simulink model "cmvk"  (R2023b)
settings: Solver=VariableStepAuto  StartTime=0.0  StopTime=700  RelTol=1e-3
settings Model: Creator=Iustin  LastModifiedBy=Iustin

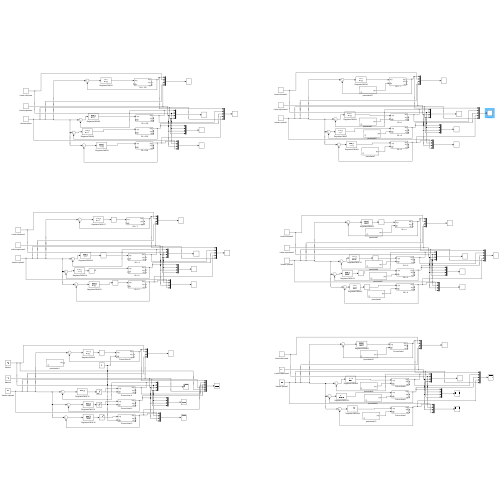
[thumbnail: Simulink's stored preview of the top-level diagram]
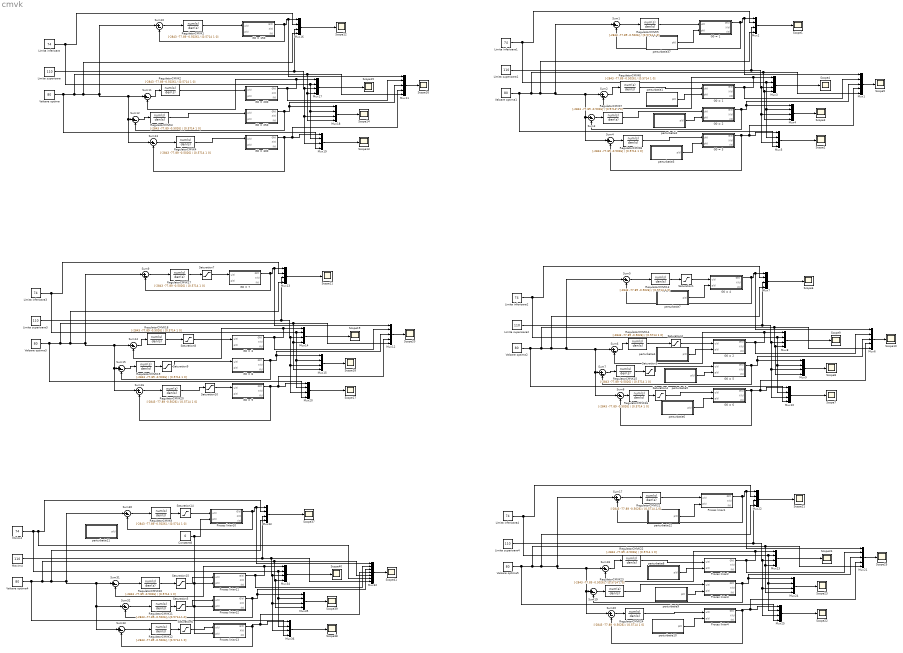
== system cmvk ==
  "  G0 = 1" : Subsystem  mask{p1=0.005, p2=0.017, p3=0.00000808, n=0.175, V=120, Gb=80, G0=100}
  "  G0 = 2" : Subsystem  mask{p1=0.005, p2=0.017, p3=0.00000808, n=0.175, V=120, Gb=80, G0=100}
  "  G0 = 200" : Subsystem  mask{p1=0.005, p2=0.017, p3=0.00000808, n=0.175, V=120, Gb=80, G0=200}
  "  G0 = 3" : Subsystem  mask{p1=0.005, p2=0.017, p3=0.00000808, n=0.175, V=120, Gb=80, G0=200}
  " G0 = 1" : Subsystem  mask{p1=0.005, p2=0.017, p3=0.00000808, n=0.175, V=120, Gb=80, G0=100}
  " G0 = 150" : Subsystem  mask{p1=0.005, p2=0.017, p3=0.00000808, n=0.175, V=120, Gb=80, G0=150}
  " G0 = 2" : Subsystem  mask{p1=0.005, p2=0.017, p3=0.00000808, n=0.175, V=120, Gb=80, G0=100}
  " G0 = 250" : Subsystem  mask{p1=0.005, p2=0.017, p3=0.00000808, n=0.175, V=120, Gb=80, G0=250}
  " G0 = 3" : Subsystem  mask{p1=0.005, p2=0.017, p3=0.00000808, n=0.175, V=120, Gb=80, G0=100}
  " G0 = 300" : Subsystem  mask{p1=0.005, p2=0.017, p3=0.00000808, n=0.175, V=120, Gb=80, G0=300}
  " G0 = 4" : Subsystem  mask{p1=0.005, p2=0.017, p3=0.00000808, n=0.175, V=120, Gb=80, G0=100}
  " G0 = 5" : Subsystem  mask{p1=0.005, p2=0.017, p3=0.00000808, n=0.175, V=120, Gb=80, G0=100}
  " G0 = 6" : Subsystem  mask{p1=0.005, p2=0.017, p3=0.00000808, n=0.175, V=120, Gb=80, G0=100}
  " G0 = 7" : Subsystem  mask{p1=0.005, p2=0.017, p3=0.00000808, n=0.175, V=120, Gb=80, G0=150}
  " G0 = 8" : Subsystem  mask{p1=0.005, p2=0.017, p3=0.00000808, n=0.175, V=120, Gb=80, G0=250}
  " G0 = 9" : Subsystem  mask{p1=0.005, p2=0.017, p3=0.00000808, n=0.175, V=120, Gb=80, G0=300}
  " Proces liniar1" : Subsystem  mask{p1=0.005, p2=0.017, p3=0.00000808, n=0.175, V=120, Gb=80, G0=150, Xb=0.0054}
  " Proces liniar10" : Subsystem  mask{p1=0.005, p2=0.017, p3=0.00000808, n=0.175, V=120, Gb=80, G0=150, Xb=0.0054}
  " Proces liniar11" : Subsystem  mask{p1=0.005, p2=0.017, p3=0.00000808, n=0.175, V=120, Gb=80, G0=200, Xb=0.0054}
  " Proces liniar12" : Subsystem  mask{p1=0.005, p2=0.017, p3=0.00000808, n=0.175, V=120, Gb=80, G0=250, Xb=0.0054}
  " Proces liniar13" : Subsystem  mask{p1=0.005, p2=0.017, p3=0.00000808, n=0.175, V=120, Gb=80, G0=300, Xb=0.0054}
  " Proces liniar2" : Subsystem  mask{p1=0.005, p2=0.017, p3=0.00000808, n=0.175, V=120, Gb=80, G0=150, Xb=0.0054}
  " Proces liniar3" : Subsystem  mask{p1=0.005, p2=0.017, p3=0.00000808, n=0.175, V=120, Gb=80, G0=150, Xb=0.0054}
  " Proces liniar4" : Subsystem  mask{p1=0.005, p2=0.017, p3=0.00000808, n=0.175, V=120, Gb=80, G0=150, Xb=0.0054}
   RegulatorCMVK{1..24} (24 alike) : TransferFcn  Numerator=[-2843 -77.89 -0.5026]  Denominator=[0.5714 1 0]
  Constant8 : Constant  Value=0
  Limita inferioara{,1..4} (5 alike) : Constant  Value=74
  Limita superioara{,1..4} (5 alike) : Constant  Value=110
  Maxim4 : Constant  Value=110
  Minim4 : Constant  Value=74
  Mux{1,6,11..12,21} (5 alike) : Mux  Inputs=5
  Mux{2..5,7..10,13..20,22..25,33..36} (24 alike) : Mux
  Mux32 : Mux  Inputs=7
  Saturation{1..10,14..15} (12 alike) : Saturate  UpperLimit=0  LowerLimit=-500
  Scope{1..25,37..41} (30 alike) : Scope
  Sum{1..20,30..33} (24 alike) : Sum  Inputs=|+-
  Valoare optima{,1..5} (6 alike) : Constant  Value=80
  perturbatie1 : Subsystem  mask{Dg=40*1000, Ag=0.8, tg_max=40}
  perturbatie10 : Subsystem  mask{Dg=100*1000, Ag=0.8, tg_max=40}
  perturbatie11 : Subsystem  mask{Dg=100000, Ag=0.8, tg_max=40}
  perturbatie12 : Subsystem  mask{Dg=10*1000, Ag=0.8, tg_max=40}
  perturbatie2 : Subsystem  mask{Dg=70*1000, Ag=0.8, tg_max=40}
  perturbatie3 : Subsystem  mask{Dg=100*1000, Ag=0.8, tg_max=40}
  perturbatie37 : Subsystem  mask{Dg=10*1000, Ag=0.8, tg_max=40}
  perturbatie4 : Subsystem  mask{Dg=40*1000, Ag=0.8, tg_max=40}
  perturbatie5 : Subsystem  mask{Dg=70*1000, Ag=0.8, tg_max=40}
  perturbatie6 : Subsystem  mask{Dg=100*1000, Ag=0.8, tg_max=40}
  perturbatie7 : Subsystem  mask{Dg=10*1000, Ag=0.8, tg_max=40}
  perturbatie8 : Subsystem  mask{Dg=40*1000, Ag=0.8, tg_max=40}
  perturbatie9 : Subsystem  mask{Dg=70*1000, Ag=0.8, tg_max=40}
  wires:
  Saturation4/1 -> " G0 = 6"/1(" u(t)")
  " G0 = 5"/1(" G(t)") -> Mux6/3, Mux9/1, Sum7/2
  perturbatie4/1(p(t)) -> "  G0 = 2"/2(p(t))
  perturbatie6/1(p(t)) -> " G0 = 6"/2(p(t))
  Mux6/1 -> Scope10/1
  Sum6/1 -> " RegulatorCMVK14"/1
  " RegulatorCMVK15"/1 -> Saturation3/1
  Mux8/1 -> Scope9/1
  Sum5/1 -> " RegulatorCMVK13"/1
  Mux10/1 -> Scope7/1
  " RegulatorCMVK16"/1 -> Saturation4/1
  perturbatie5/1(p(t)) -> " G0 = 5"/2(p(t))
  Limita inferioara2/1 -> Mux10/2, Mux9/2, Mux8/2, Mux7/2
  Sum8/1 -> " RegulatorCMVK16"/1
  Sum30/1 -> " RegulatorCMVK9"/1
  Saturation6/1 -> " Proces liniar13"/1(" u(t)")
  Constant8/1 -> " Proces liniar10"/2(p(t)), " Proces liniar11"/2(p(t)), " Proces liniar13"/2(p(t)), " Proces liniar12"/2(p(t))
  " Proces liniar13"/1(" G(t)") -> Mux32/4, Mux36/1, Sum33/2
  Mux35/1 -> Scope39/1
  Sum31/1 -> " RegulatorCMVK10"/1
  Valoare optima4/1 -> Mux36/4, Mux35/4, Mux34/4, Mux32/5, Mux33/4, Sum30/1, Sum33/1, Sum32/1, Sum31/1
  Mux33/1 -> Scope37/1
  Mux32/1 -> Scope41/1
  " RegulatorCMVK12"/1 -> Saturation6/1
  " RegulatorCMVK13"/1 -> Saturation1/1
  Maxim4/1 -> Mux32/7, Mux36/3, Mux35/3, Mux34/3, Mux33/3
  Saturation5/1 -> " Proces liniar12"/1(" u(t)")
  " G0 = 6"/1(" G(t)") -> Mux6/4, Mux10/1, Sum8/2
  perturbatie7/1(p(t)) -> " G0 = 4"/2(p(t))
  Saturation14/1 -> " Proces liniar10"/1(" u(t)")
  Saturation15/1 -> " Proces liniar11"/1(" u(t)")
  Sum32/1 -> " RegulatorCMVK11"/1
  Sum33/1 -> " RegulatorCMVK12"/1
  Saturation2/1 -> "  G0 = 2"/1(" u(t)")
  " RegulatorCMVK11"/1 -> Saturation5/1
  " RegulatorCMVK2"/1 -> "  G0 = 200"/1(" u(t)")
  " Proces liniar10"/1(" G(t)") -> Sum30/2, Mux32/1, Mux33/1
  Sum12/1 -> " RegulatorCMVK3"/1
  " G0 = 150"/1(" G(t)") -> Sum10/2, Mux11/1, Mux16/1
  " Proces liniar11"/1(" G(t)") -> Mux32/2, Mux34/1, Sum31/2
  " RegulatorCMVK8"/1 -> " G0 = 3"/1(" u(t)")
  Mux7/1 -> Scope6/1
  " G0 = 3"/1(" G(t)") -> Mux1/4, Mux5/1, Sum4/2
  Mux4/1 -> Scope3/1
  Limita superioara1/1 -> Mux5/3, Mux4/3, Mux3/3, Mux2/3
  " G0 = 2"/1(" G(t)") -> Mux1/3, Mux4/1, Sum3/2
  Sum4/1 -> " RegulatorCMVK8"/1
  Sum11/1 -> " RegulatorCMVK2"/1
  "  G0 = 1"/1(" G(t)") -> Mux1/2, Mux3/1, Sum2/2
  Sum1/1 -> " RegulatorCMVK5"/1
  " RegulatorCMVK10"/1 -> Saturation15/1
  " G0 = 1"/1(" G(t)") -> Sum1/2, Mux1/1, Mux2/1
  "  G0 = 200"/1(" G(t)") -> Mux11/2, Mux17/1, Sum11/2
  Sum3/1 -> " RegulatorCMVK7"/1
  Mux5/1 -> Scope2/1
  Mux1/1 -> Scope5/1
  " G0 = 4"/1(" G(t)") -> Sum5/2, Mux6/1, Mux7/1
  " RegulatorCMVK14"/1 -> Saturation2/1
  " RegulatorCMVK9"/1 -> Saturation14/1
  Valoare optima1/1 -> Mux5/4, Mux4/4, Mux3/4, Mux1/5, Mux2/4, Sum1/1, Sum4/1, Sum3/1, Sum2/1
  " RegulatorCMVK7"/1 -> " G0 = 2"/1(" u(t)")
  Valoare optima2/1 -> Mux10/4, Mux9/4, Mux8/4, Mux6/5, Mux7/4, Sum5/1, Sum8/1, Sum7/1, Sum6/1
  perturbatie1/1(p(t)) -> "  G0 = 1"/2(p(t))
  Mux11/1 -> Scope16/1
  "  G0 = 2"/1(" G(t)") -> Mux6/2, Mux8/1, Sum6/2
  Sum10/1 -> " RegulatorCMVK1"/1
  Mux34/1 -> Scope40/1
  Mux19/1 -> Scope13/1
  Sum2/1 -> " RegulatorCMVK6"/1
  " RegulatorCMVK3"/1 -> " G0 = 250"/1(" u(t)")
  Limita superioara/1 -> Mux19/3, Mux18/3, Mux17/3, Mux16/3
  Mux36/1 -> Scope38/1
  Mux3/1 -> Scope4/1
  " RegulatorCMVK6"/1 -> "  G0 = 1"/1(" u(t)")
  " Proces liniar12"/1(" G(t)") -> Mux32/3, Mux35/1, Sum32/2
  Mux2/1 -> Scope1/1
  Saturation3/1 -> " G0 = 5"/1(" u(t)")
  Mux16/1 -> Scope12/1
  " G0 = 250"/1(" G(t)") -> Mux11/3, Mux18/1, Sum12/2
  Mux18/1 -> Scope14/1
  Sum13/1 -> " RegulatorCMVK4"/1
  " G0 = 300"/1(" G(t)") -> Mux11/4, Mux19/1, Sum13/2
  Minim4/1 -> Mux36/2, Mux35/2, Mux34/2, Mux32/6, Mux33/2
  " RegulatorCMVK4"/1 -> " G0 = 300"/1(" u(t)")
  Limita inferioara/1 -> Mux19/2, Mux18/2, Mux17/2, Mux16/2
  " RegulatorCMVK5"/1 -> " G0 = 1"/1(" u(t)")
  perturbatie2/1(p(t)) -> " G0 = 2"/2(p(t))
  " RegulatorCMVK1"/1 -> " G0 = 150"/1(" u(t)")
  Limita superioara2/1 -> Mux10/3, Mux9/3, Mux8/3, Mux7/3
  Mux9/1 -> Scope8/1
  Limita inferioara1/1 -> Mux5/2, Mux4/2, Mux3/2, Mux2/2
  Valoare optima/1 -> Mux19/4, Mux18/4, Mux17/4, Mux11/5, Mux16/4, Sum10/1, Sum13/1, Sum12/1, Sum11/1
  perturbatie37/1(p(t)) -> " G0 = 1"/2(p(t))
  Sum7/1 -> " RegulatorCMVK15"/1
  Mux17/1 -> Scope15/1
  Saturation1/1 -> " G0 = 4"/1(" u(t)")
  perturbatie3/1(p(t)) -> " G0 = 3"/2(p(t))
  " RegulatorCMVK20"/1 -> Saturation10/1
  Sum9/1 -> " RegulatorCMVK17"/1
  " RegulatorCMVK19"/1 -> Saturation9/1
  Mux13/1 -> Scope11/1
  "  G0 = 3"/1(" G(t)") -> Mux12/2, Mux14/1, Sum14/2
  Limita superioara3/1 -> Mux20/3, Mux15/3, Mux14/3, Mux13/3
  " RegulatorCMVK17"/1 -> Saturation7/1
  Sum15/1 -> " RegulatorCMVK19"/1
  Sum14/1 -> " RegulatorCMVK18"/1
  " RegulatorCMVK18"/1 -> Saturation8/1
  Limita inferioara3/1 -> Mux20/2, Mux15/2, Mux14/2, Mux13/2
  Mux14/1 -> Scope19/1
  Mux20/1 -> Scope17/1
  Sum16/1 -> " RegulatorCMVK20"/1
  Mux15/1 -> Scope18/1
  Mux12/1 -> Scope20/1
  " G0 = 8"/1(" G(t)") -> Mux12/3, Mux15/1, Sum15/2
  Valoare optima3/1 -> Mux20/4, Mux15/4, Mux14/4, Mux12/5, Mux13/4, Sum9/1, Sum16/1, Sum15/1, Sum14/1
  " G0 = 9"/1(" G(t)") -> Mux12/4, Mux20/1, Sum16/2
  " G0 = 7"/1(" G(t)") -> Sum9/2, Mux12/1, Mux13/1
  Saturation7/1 -> " G0 = 7"/1(" u(t)")
  Saturation8/1 -> "  G0 = 3"/1(" u(t)")
  Saturation9/1 -> " G0 = 8"/1(" u(t)")
  Saturation10/1 -> " G0 = 9"/1(" u(t)")
  " RegulatorCMVK24"/1 -> " Proces liniar4"/1(" u(t)")
  Limita inferioara4/1 -> Mux25/2, Mux24/2, Mux23/2, Mux22/2
  Mux25/1 -> Scope22/1
  Sum20/1 -> " RegulatorCMVK24"/1
  Sum17/1 -> " RegulatorCMVK21"/1
  Mux22/1 -> Scope21/1
  " RegulatorCMVK22"/1 -> " Proces liniar2"/1(" u(t)")
  Sum19/1 -> " RegulatorCMVK23"/1
  Limita superioara4/1 -> Mux25/3, Mux24/3, Mux23/3, Mux22/3
  Mux24/1 -> Scope23/1
  " RegulatorCMVK23"/1 -> " Proces liniar3"/1(" u(t)")
  perturbatie8/1(p(t)) -> " Proces liniar2"/2(p(t))
  perturbatie9/1(p(t)) -> " Proces liniar3"/2(p(t))
  " Proces liniar4"/1(" G(t)") -> Mux21/4, Mux25/1, Sum20/2
  " Proces liniar1"/1(" G(t)") -> Sum17/2, Mux21/1, Mux22/1
  Sum18/1 -> " RegulatorCMVK22"/1
  Mux21/1 -> Scope25/1
  " Proces liniar2"/1(" G(t)") -> Mux21/2, Mux23/1, Sum18/2
  Valoare optima5/1 -> Mux25/4, Mux24/4, Mux23/4, Mux21/5, Mux22/4, Sum17/1, Sum20/1, Sum19/1, Sum18/1
  " RegulatorCMVK21"/1 -> " Proces liniar1"/1(" u(t)")
  Mux23/1 -> Scope24/1
  perturbatie10/1(p(t)) -> " Proces liniar4"/2(p(t))
  " Proces liniar3"/1(" G(t)") -> Mux21/3, Mux24/1, Sum19/2
  perturbatie12/1(p(t)) -> " Proces liniar1"/2(p(t))

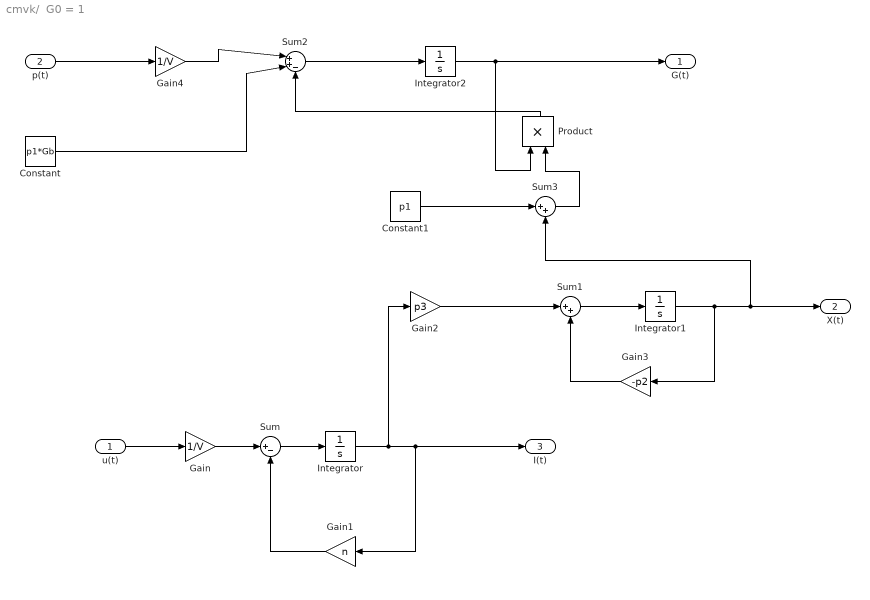
== system cmvk/  G0 = 1 ==
  " u(t)" : Inport
  p(t) : Inport  Port=2
  Constant : Constant  Value=p1*Gb
  Constant1 : Constant  Value=p1
  Gain : Gain  Gain=1/V
  Gain1 : Gain  Gain=n
  Gain2 : Gain  Gain=p3
  Gain3 : Gain  Gain=-p2
  Gain4 : Gain  Gain=1/V
  Integrator : Integrator
  Integrator1 : Integrator
  Integrator2 : Integrator  InitialCondition=G0
  Product : Product
  Sum : Sum  Inputs=|+-
  Sum1 : Sum  Inputs=|++
  Sum2 : Sum  Inputs=|++-
  Sum3 : Sum  Inputs=|++
  " G(t)" : Outport
  X(t) : Outport  Port=2
  I(t) : Outport  Port=3
  wires:
  " u(t)"/1 -> Gain/1
  Gain/1 -> Sum/1
  Sum/1 -> Integrator/1
  Integrator/1 -> Gain2/1, I(t)/1, Gain1/1
  Gain1/1 -> Sum/2
  Gain2/1 -> Sum1/1
  Gain3/1 -> Sum1/2
  Integrator1/1 -> Gain3/1, Sum3/2, X(t)/1
  p(t)/1 -> Gain4/1
  Gain4/1 -> Sum2/1
  Constant/1 -> Sum2/2
  Constant1/1 -> Sum3/1
  Sum2/1 -> Integrator2/1
  Product/1 -> Sum2/3
  Sum3/1 -> Product/2
  Integrator2/1 -> Product/1, " G(t)"/1
  Sum1/1 -> Integrator1/1

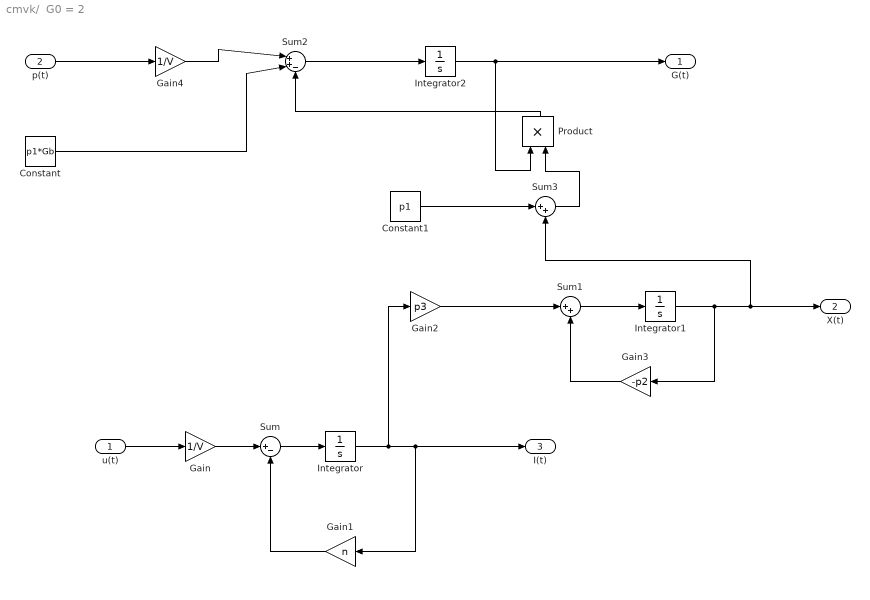
== system cmvk/  G0 = 2 ==
  " u(t)" : Inport
  p(t) : Inport  Port=2
  Constant : Constant  Value=p1*Gb
  Constant1 : Constant  Value=p1
  Gain : Gain  Gain=1/V
  Gain1 : Gain  Gain=n
  Gain2 : Gain  Gain=p3
  Gain3 : Gain  Gain=-p2
  Gain4 : Gain  Gain=1/V
  Integrator : Integrator
  Integrator1 : Integrator
  Integrator2 : Integrator  InitialCondition=G0
  Product : Product
  Sum : Sum  Inputs=|+-
  Sum1 : Sum  Inputs=|++
  Sum2 : Sum  Inputs=|++-
  Sum3 : Sum  Inputs=|++
  " G(t)" : Outport
  X(t) : Outport  Port=2
  I(t) : Outport  Port=3
  wires:
  " u(t)"/1 -> Gain/1
  Gain/1 -> Sum/1
  Sum/1 -> Integrator/1
  Integrator/1 -> Gain2/1, I(t)/1, Gain1/1
  Gain1/1 -> Sum/2
  Gain2/1 -> Sum1/1
  Gain3/1 -> Sum1/2
  Integrator1/1 -> Gain3/1, Sum3/2, X(t)/1
  p(t)/1 -> Gain4/1
  Gain4/1 -> Sum2/1
  Constant/1 -> Sum2/2
  Constant1/1 -> Sum3/1
  Sum2/1 -> Integrator2/1
  Product/1 -> Sum2/3
  Sum3/1 -> Product/2
  Integrator2/1 -> Product/1, " G(t)"/1
  Sum1/1 -> Integrator1/1

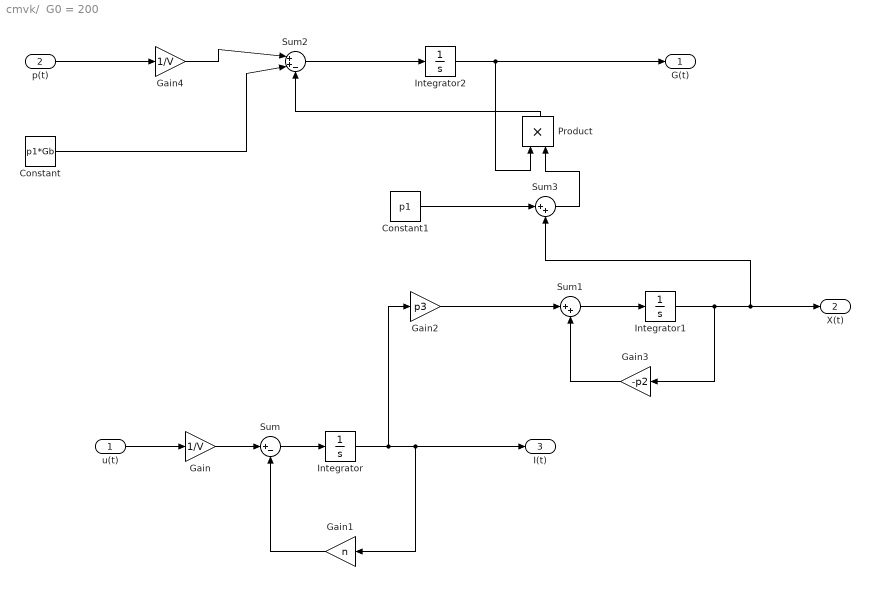
== system cmvk/  G0 = 200 ==
  " u(t)" : Inport
  p(t) : Inport  Port=2
  Constant : Constant  Value=p1*Gb
  Constant1 : Constant  Value=p1
  Gain : Gain  Gain=1/V
  Gain1 : Gain  Gain=n
  Gain2 : Gain  Gain=p3
  Gain3 : Gain  Gain=-p2
  Gain4 : Gain  Gain=1/V
  Integrator : Integrator
  Integrator1 : Integrator
  Integrator2 : Integrator  InitialCondition=G0
  Product : Product
  Sum : Sum  Inputs=|+-
  Sum1 : Sum  Inputs=|++
  Sum2 : Sum  Inputs=|++-
  Sum3 : Sum  Inputs=|++
  " G(t)" : Outport
  X(t) : Outport  Port=2
  I(t) : Outport  Port=3
  wires:
  " u(t)"/1 -> Gain/1
  Gain/1 -> Sum/1
  Sum/1 -> Integrator/1
  Integrator/1 -> Gain2/1, I(t)/1, Gain1/1
  Gain1/1 -> Sum/2
  Gain2/1 -> Sum1/1
  Gain3/1 -> Sum1/2
  Integrator1/1 -> Gain3/1, Sum3/2, X(t)/1
  p(t)/1 -> Gain4/1
  Gain4/1 -> Sum2/1
  Constant/1 -> Sum2/2
  Constant1/1 -> Sum3/1
  Sum2/1 -> Integrator2/1
  Product/1 -> Sum2/3
  Sum3/1 -> Product/2
  Integrator2/1 -> Product/1, " G(t)"/1
  Sum1/1 -> Integrator1/1

== system cmvk/  G0 = 3 ==
  " u(t)" : Inport
  p(t) : Inport  Port=2
  Constant : Constant  Value=p1*Gb
  Constant1 : Constant  Value=p1
  Gain : Gain  Gain=1/V
  Gain1 : Gain  Gain=n
  Gain2 : Gain  Gain=p3
  Gain3 : Gain  Gain=-p2
  Gain4 : Gain  Gain=1/V
  Integrator : Integrator
  Integrator1 : Integrator
  Integrator2 : Integrator  InitialCondition=G0
  Product : Product
  Sum : Sum  Inputs=|+-
  Sum1 : Sum  Inputs=|++
  Sum2 : Sum  Inputs=|++-
  Sum3 : Sum  Inputs=|++
  " G(t)" : Outport
  X(t) : Outport  Port=2
  I(t) : Outport  Port=3
  wires:
  " u(t)"/1 -> Gain/1
  Gain/1 -> Sum/1
  Sum/1 -> Integrator/1
  Integrator/1 -> Gain2/1, I(t)/1, Gain1/1
  Gain1/1 -> Sum/2
  Gain2/1 -> Sum1/1
  Gain3/1 -> Sum1/2
  Integrator1/1 -> Gain3/1, Sum3/2, X(t)/1
  p(t)/1 -> Gain4/1
  Gain4/1 -> Sum2/1
  Constant/1 -> Sum2/2
  Constant1/1 -> Sum3/1
  Sum2/1 -> Integrator2/1
  Product/1 -> Sum2/3
  Sum3/1 -> Product/2
  Integrator2/1 -> Product/1, " G(t)"/1
  Sum1/1 -> Integrator1/1

== system cmvk/ G0 = 1 ==
  " u(t)" : Inport
  p(t) : Inport  Port=2
  Constant : Constant  Value=p1*Gb
  Constant1 : Constant  Value=p1
  Gain : Gain  Gain=1/V
  Gain1 : Gain  Gain=n
  Gain2 : Gain  Gain=p3
  Gain3 : Gain  Gain=-p2
  Gain4 : Gain  Gain=1/V
  Integrator : Integrator
  Integrator1 : Integrator
  Integrator2 : Integrator  InitialCondition=G0
  Product : Product
  Sum : Sum  Inputs=|+-
  Sum1 : Sum  Inputs=|++
  Sum2 : Sum  Inputs=|++-
  Sum3 : Sum  Inputs=|++
  " G(t)" : Outport
  X(t) : Outport  Port=2
  I(t) : Outport  Port=3
  wires:
  " u(t)"/1 -> Gain/1
  Gain/1 -> Sum/1
  Sum/1 -> Integrator/1
  Integrator/1 -> Gain2/1, I(t)/1, Gain1/1
  Gain1/1 -> Sum/2
  Gain2/1 -> Sum1/1
  Gain3/1 -> Sum1/2
  Integrator1/1 -> Gain3/1, Sum3/2, X(t)/1
  p(t)/1 -> Gain4/1
  Gain4/1 -> Sum2/1
  Constant/1 -> Sum2/2
  Constant1/1 -> Sum3/1
  Sum2/1 -> Integrator2/1
  Product/1 -> Sum2/3
  Sum3/1 -> Product/2
  Integrator2/1 -> Product/1, " G(t)"/1
  Sum1/1 -> Integrator1/1

== system cmvk/ G0 = 150 ==
  " u(t)" : Inport
  p(t) : Inport  Port=2
  Constant : Constant  Value=p1*Gb
  Constant1 : Constant  Value=p1
  Gain : Gain  Gain=1/V
  Gain1 : Gain  Gain=n
  Gain2 : Gain  Gain=p3
  Gain3 : Gain  Gain=-p2
  Gain4 : Gain  Gain=1/V
  Integrator : Integrator
  Integrator1 : Integrator
  Integrator2 : Integrator  InitialCondition=G0
  Product : Product
  Sum : Sum  Inputs=|+-
  Sum1 : Sum  Inputs=|++
  Sum2 : Sum  Inputs=|++-
  Sum3 : Sum  Inputs=|++
  " G(t)" : Outport
  X(t) : Outport  Port=2
  I(t) : Outport  Port=3
  wires:
  " u(t)"/1 -> Gain/1
  Gain/1 -> Sum/1
  Sum/1 -> Integrator/1
  Integrator/1 -> Gain2/1, I(t)/1, Gain1/1
  Gain1/1 -> Sum/2
  Gain2/1 -> Sum1/1
  Gain3/1 -> Sum1/2
  Integrator1/1 -> Gain3/1, Sum3/2, X(t)/1
  p(t)/1 -> Gain4/1
  Gain4/1 -> Sum2/1
  Constant/1 -> Sum2/2
  Constant1/1 -> Sum3/1
  Sum2/1 -> Integrator2/1
  Product/1 -> Sum2/3
  Sum3/1 -> Product/2
  Integrator2/1 -> Product/1, " G(t)"/1
  Sum1/1 -> Integrator1/1

== system cmvk/ G0 = 2 ==
  " u(t)" : Inport
  p(t) : Inport  Port=2
  Constant : Constant  Value=p1*Gb
  Constant1 : Constant  Value=p1
  Gain : Gain  Gain=1/V
  Gain1 : Gain  Gain=n
  Gain2 : Gain  Gain=p3
  Gain3 : Gain  Gain=-p2
  Gain4 : Gain  Gain=1/V
  Integrator : Integrator
  Integrator1 : Integrator
  Integrator2 : Integrator  InitialCondition=G0
  Product : Product
  Sum : Sum  Inputs=|+-
  Sum1 : Sum  Inputs=|++
  Sum2 : Sum  Inputs=|++-
  Sum3 : Sum  Inputs=|++
  " G(t)" : Outport
  X(t) : Outport  Port=2
  I(t) : Outport  Port=3
  wires:
  " u(t)"/1 -> Gain/1
  Gain/1 -> Sum/1
  Sum/1 -> Integrator/1
  Integrator/1 -> Gain2/1, I(t)/1, Gain1/1
  Gain1/1 -> Sum/2
  Gain2/1 -> Sum1/1
  Gain3/1 -> Sum1/2
  Integrator1/1 -> Gain3/1, Sum3/2, X(t)/1
  p(t)/1 -> Gain4/1
  Gain4/1 -> Sum2/1
  Constant/1 -> Sum2/2
  Constant1/1 -> Sum3/1
  Sum2/1 -> Integrator2/1
  Product/1 -> Sum2/3
  Sum3/1 -> Product/2
  Integrator2/1 -> Product/1, " G(t)"/1
  Sum1/1 -> Integrator1/1

== system cmvk/ G0 = 250 ==
  " u(t)" : Inport
  p(t) : Inport  Port=2
  Constant : Constant  Value=p1*Gb
  Constant1 : Constant  Value=p1
  Gain : Gain  Gain=1/V
  Gain1 : Gain  Gain=n
  Gain2 : Gain  Gain=p3
  Gain3 : Gain  Gain=-p2
  Gain4 : Gain  Gain=1/V
  Integrator : Integrator
  Integrator1 : Integrator
  Integrator2 : Integrator  InitialCondition=G0
  Product : Product
  Sum : Sum  Inputs=|+-
  Sum1 : Sum  Inputs=|++
  Sum2 : Sum  Inputs=|++-
  Sum3 : Sum  Inputs=|++
  " G(t)" : Outport
  X(t) : Outport  Port=2
  I(t) : Outport  Port=3
  wires:
  " u(t)"/1 -> Gain/1
  Gain/1 -> Sum/1
  Sum/1 -> Integrator/1
  Integrator/1 -> Gain2/1, I(t)/1, Gain1/1
  Gain1/1 -> Sum/2
  Gain2/1 -> Sum1/1
  Gain3/1 -> Sum1/2
  Integrator1/1 -> Gain3/1, Sum3/2, X(t)/1
  p(t)/1 -> Gain4/1
  Gain4/1 -> Sum2/1
  Constant/1 -> Sum2/2
  Constant1/1 -> Sum3/1
  Sum2/1 -> Integrator2/1
  Product/1 -> Sum2/3
  Sum3/1 -> Product/2
  Integrator2/1 -> Product/1, " G(t)"/1
  Sum1/1 -> Integrator1/1

== system cmvk/ G0 = 3 ==
  " u(t)" : Inport
  p(t) : Inport  Port=2
  Constant : Constant  Value=p1*Gb
  Constant1 : Constant  Value=p1
  Gain : Gain  Gain=1/V
  Gain1 : Gain  Gain=n
  Gain2 : Gain  Gain=p3
  Gain3 : Gain  Gain=-p2
  Gain4 : Gain  Gain=1/V
  Integrator : Integrator
  Integrator1 : Integrator
  Integrator2 : Integrator  InitialCondition=G0
  Product : Product
  Sum : Sum  Inputs=|+-
  Sum1 : Sum  Inputs=|++
  Sum2 : Sum  Inputs=|++-
  Sum3 : Sum  Inputs=|++
  " G(t)" : Outport
  X(t) : Outport  Port=2
  I(t) : Outport  Port=3
  wires:
  " u(t)"/1 -> Gain/1
  Gain/1 -> Sum/1
  Sum/1 -> Integrator/1
  Integrator/1 -> Gain2/1, I(t)/1, Gain1/1
  Gain1/1 -> Sum/2
  Gain2/1 -> Sum1/1
  Gain3/1 -> Sum1/2
  Integrator1/1 -> Gain3/1, Sum3/2, X(t)/1
  p(t)/1 -> Gain4/1
  Gain4/1 -> Sum2/1
  Constant/1 -> Sum2/2
  Constant1/1 -> Sum3/1
  Sum2/1 -> Integrator2/1
  Product/1 -> Sum2/3
  Sum3/1 -> Product/2
  Integrator2/1 -> Product/1, " G(t)"/1
  Sum1/1 -> Integrator1/1

== system cmvk/ G0 = 300 ==
  " u(t)" : Inport
  p(t) : Inport  Port=2
  Constant : Constant  Value=p1*Gb
  Constant1 : Constant  Value=p1
  Gain : Gain  Gain=1/V
  Gain1 : Gain  Gain=n
  Gain2 : Gain  Gain=p3
  Gain3 : Gain  Gain=-p2
  Gain4 : Gain  Gain=1/V
  Integrator : Integrator
  Integrator1 : Integrator
  Integrator2 : Integrator  InitialCondition=G0
  Product : Product
  Sum : Sum  Inputs=|+-
  Sum1 : Sum  Inputs=|++
  Sum2 : Sum  Inputs=|++-
  Sum3 : Sum  Inputs=|++
  " G(t)" : Outport
  X(t) : Outport  Port=2
  I(t) : Outport  Port=3
  wires:
  " u(t)"/1 -> Gain/1
  Gain/1 -> Sum/1
  Sum/1 -> Integrator/1
  Integrator/1 -> Gain2/1, I(t)/1, Gain1/1
  Gain1/1 -> Sum/2
  Gain2/1 -> Sum1/1
  Gain3/1 -> Sum1/2
  Integrator1/1 -> Gain3/1, Sum3/2, X(t)/1
  p(t)/1 -> Gain4/1
  Gain4/1 -> Sum2/1
  Constant/1 -> Sum2/2
  Constant1/1 -> Sum3/1
  Sum2/1 -> Integrator2/1
  Product/1 -> Sum2/3
  Sum3/1 -> Product/2
  Integrator2/1 -> Product/1, " G(t)"/1
  Sum1/1 -> Integrator1/1

== system cmvk/ G0 = 4 ==
  " u(t)" : Inport
  p(t) : Inport  Port=2
  Constant : Constant  Value=p1*Gb
  Constant1 : Constant  Value=p1
  Gain : Gain  Gain=1/V
  Gain1 : Gain  Gain=n
  Gain2 : Gain  Gain=p3
  Gain3 : Gain  Gain=-p2
  Gain4 : Gain  Gain=1/V
  Integrator : Integrator
  Integrator1 : Integrator
  Integrator2 : Integrator  InitialCondition=G0
  Product : Product
  Sum : Sum  Inputs=|+-
  Sum1 : Sum  Inputs=|++
  Sum2 : Sum  Inputs=|++-
  Sum3 : Sum  Inputs=|++
  " G(t)" : Outport
  X(t) : Outport  Port=2
  I(t) : Outport  Port=3
  wires:
  " u(t)"/1 -> Gain/1
  Gain/1 -> Sum/1
  Sum/1 -> Integrator/1
  Integrator/1 -> Gain2/1, I(t)/1, Gain1/1
  Gain1/1 -> Sum/2
  Gain2/1 -> Sum1/1
  Gain3/1 -> Sum1/2
  Integrator1/1 -> Gain3/1, Sum3/2, X(t)/1
  p(t)/1 -> Gain4/1
  Gain4/1 -> Sum2/1
  Constant/1 -> Sum2/2
  Constant1/1 -> Sum3/1
  Sum2/1 -> Integrator2/1
  Product/1 -> Sum2/3
  Sum3/1 -> Product/2
  Integrator2/1 -> Product/1, " G(t)"/1
  Sum1/1 -> Integrator1/1

== system cmvk/ G0 = 5 ==
  " u(t)" : Inport
  p(t) : Inport  Port=2
  Constant : Constant  Value=p1*Gb
  Constant1 : Constant  Value=p1
  Gain : Gain  Gain=1/V
  Gain1 : Gain  Gain=n
  Gain2 : Gain  Gain=p3
  Gain3 : Gain  Gain=-p2
  Gain4 : Gain  Gain=1/V
  Integrator : Integrator
  Integrator1 : Integrator
  Integrator2 : Integrator  InitialCondition=G0
  Product : Product
  Sum : Sum  Inputs=|+-
  Sum1 : Sum  Inputs=|++
  Sum2 : Sum  Inputs=|++-
  Sum3 : Sum  Inputs=|++
  " G(t)" : Outport
  X(t) : Outport  Port=2
  I(t) : Outport  Port=3
  wires:
  " u(t)"/1 -> Gain/1
  Gain/1 -> Sum/1
  Sum/1 -> Integrator/1
  Integrator/1 -> Gain2/1, I(t)/1, Gain1/1
  Gain1/1 -> Sum/2
  Gain2/1 -> Sum1/1
  Gain3/1 -> Sum1/2
  Integrator1/1 -> Gain3/1, Sum3/2, X(t)/1
  p(t)/1 -> Gain4/1
  Gain4/1 -> Sum2/1
  Constant/1 -> Sum2/2
  Constant1/1 -> Sum3/1
  Sum2/1 -> Integrator2/1
  Product/1 -> Sum2/3
  Sum3/1 -> Product/2
  Integrator2/1 -> Product/1, " G(t)"/1
  Sum1/1 -> Integrator1/1

== system cmvk/ G0 = 6 ==
  " u(t)" : Inport
  p(t) : Inport  Port=2
  Constant : Constant  Value=p1*Gb
  Constant1 : Constant  Value=p1
  Gain : Gain  Gain=1/V
  Gain1 : Gain  Gain=n
  Gain2 : Gain  Gain=p3
  Gain3 : Gain  Gain=-p2
  Gain4 : Gain  Gain=1/V
  Integrator : Integrator
  Integrator1 : Integrator
  Integrator2 : Integrator  InitialCondition=G0
  Product : Product
  Sum : Sum  Inputs=|+-
  Sum1 : Sum  Inputs=|++
  Sum2 : Sum  Inputs=|++-
  Sum3 : Sum  Inputs=|++
  " G(t)" : Outport
  X(t) : Outport  Port=2
  I(t) : Outport  Port=3
  wires:
  " u(t)"/1 -> Gain/1
  Gain/1 -> Sum/1
  Sum/1 -> Integrator/1
  Integrator/1 -> Gain2/1, I(t)/1, Gain1/1
  Gain1/1 -> Sum/2
  Gain2/1 -> Sum1/1
  Gain3/1 -> Sum1/2
  Integrator1/1 -> Gain3/1, Sum3/2, X(t)/1
  p(t)/1 -> Gain4/1
  Gain4/1 -> Sum2/1
  Constant/1 -> Sum2/2
  Constant1/1 -> Sum3/1
  Sum2/1 -> Integrator2/1
  Product/1 -> Sum2/3
  Sum3/1 -> Product/2
  Integrator2/1 -> Product/1, " G(t)"/1
  Sum1/1 -> Integrator1/1

== system cmvk/ G0 = 7 ==
  " u(t)" : Inport
  p(t) : Inport  Port=2
  Constant : Constant  Value=p1*Gb
  Constant1 : Constant  Value=p1
  Gain : Gain  Gain=1/V
  Gain1 : Gain  Gain=n
  Gain2 : Gain  Gain=p3
  Gain3 : Gain  Gain=-p2
  Gain4 : Gain  Gain=1/V
  Integrator : Integrator
  Integrator1 : Integrator
  Integrator2 : Integrator  InitialCondition=G0
  Product : Product
  Sum : Sum  Inputs=|+-
  Sum1 : Sum  Inputs=|++
  Sum2 : Sum  Inputs=|++-
  Sum3 : Sum  Inputs=|++
  " G(t)" : Outport
  X(t) : Outport  Port=2
  I(t) : Outport  Port=3
  wires:
  " u(t)"/1 -> Gain/1
  Gain/1 -> Sum/1
  Sum/1 -> Integrator/1
  Integrator/1 -> Gain2/1, I(t)/1, Gain1/1
  Gain1/1 -> Sum/2
  Gain2/1 -> Sum1/1
  Gain3/1 -> Sum1/2
  Integrator1/1 -> Gain3/1, Sum3/2, X(t)/1
  p(t)/1 -> Gain4/1
  Gain4/1 -> Sum2/1
  Constant/1 -> Sum2/2
  Constant1/1 -> Sum3/1
  Sum2/1 -> Integrator2/1
  Product/1 -> Sum2/3
  Sum3/1 -> Product/2
  Integrator2/1 -> Product/1, " G(t)"/1
  Sum1/1 -> Integrator1/1

== system cmvk/ G0 = 8 ==
  " u(t)" : Inport
  p(t) : Inport  Port=2
  Constant : Constant  Value=p1*Gb
  Constant1 : Constant  Value=p1
  Gain : Gain  Gain=1/V
  Gain1 : Gain  Gain=n
  Gain2 : Gain  Gain=p3
  Gain3 : Gain  Gain=-p2
  Gain4 : Gain  Gain=1/V
  Integrator : Integrator
  Integrator1 : Integrator
  Integrator2 : Integrator  InitialCondition=G0
  Product : Product
  Sum : Sum  Inputs=|+-
  Sum1 : Sum  Inputs=|++
  Sum2 : Sum  Inputs=|++-
  Sum3 : Sum  Inputs=|++
  " G(t)" : Outport
  X(t) : Outport  Port=2
  I(t) : Outport  Port=3
  wires:
  " u(t)"/1 -> Gain/1
  Gain/1 -> Sum/1
  Sum/1 -> Integrator/1
  Integrator/1 -> Gain2/1, I(t)/1, Gain1/1
  Gain1/1 -> Sum/2
  Gain2/1 -> Sum1/1
  Gain3/1 -> Sum1/2
  Integrator1/1 -> Gain3/1, Sum3/2, X(t)/1
  p(t)/1 -> Gain4/1
  Gain4/1 -> Sum2/1
  Constant/1 -> Sum2/2
  Constant1/1 -> Sum3/1
  Sum2/1 -> Integrator2/1
  Product/1 -> Sum2/3
  Sum3/1 -> Product/2
  Integrator2/1 -> Product/1, " G(t)"/1
  Sum1/1 -> Integrator1/1

== system cmvk/ G0 = 9 ==
  " u(t)" : Inport
  p(t) : Inport  Port=2
  Constant : Constant  Value=p1*Gb
  Constant1 : Constant  Value=p1
  Gain : Gain  Gain=1/V
  Gain1 : Gain  Gain=n
  Gain2 : Gain  Gain=p3
  Gain3 : Gain  Gain=-p2
  Gain4 : Gain  Gain=1/V
  Integrator : Integrator
  Integrator1 : Integrator
  Integrator2 : Integrator  InitialCondition=G0
  Product : Product
  Sum : Sum  Inputs=|+-
  Sum1 : Sum  Inputs=|++
  Sum2 : Sum  Inputs=|++-
  Sum3 : Sum  Inputs=|++
  " G(t)" : Outport
  X(t) : Outport  Port=2
  I(t) : Outport  Port=3
  wires:
  " u(t)"/1 -> Gain/1
  Gain/1 -> Sum/1
  Sum/1 -> Integrator/1
  Integrator/1 -> Gain2/1, I(t)/1, Gain1/1
  Gain1/1 -> Sum/2
  Gain2/1 -> Sum1/1
  Gain3/1 -> Sum1/2
  Integrator1/1 -> Gain3/1, Sum3/2, X(t)/1
  p(t)/1 -> Gain4/1
  Gain4/1 -> Sum2/1
  Constant/1 -> Sum2/2
  Constant1/1 -> Sum3/1
  Sum2/1 -> Integrator2/1
  Product/1 -> Sum2/3
  Sum3/1 -> Product/2
  Integrator2/1 -> Product/1, " G(t)"/1
  Sum1/1 -> Integrator1/1

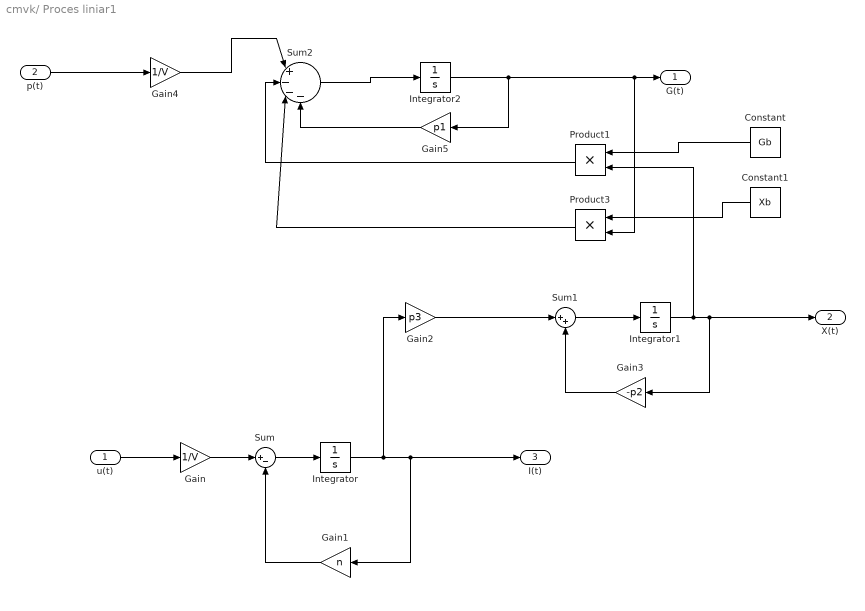
== system cmvk/ Proces liniar1 ==
  " u(t)" : Inport
  p(t) : Inport  Port=2
  Constant : Constant  Value=Gb
  Constant1 : Constant  Value=Xb
  Gain : Gain  Gain=1/V
  Gain1 : Gain  Gain=n
  Gain2 : Gain  Gain=p3
  Gain3 : Gain  Gain=-p2
  Gain4 : Gain  Gain=1/V
  Gain5 : Gain  Gain=p1
  Integrator : Integrator
  Integrator1 : Integrator
  Integrator2 : Integrator  InitialCondition=G0
  Product1 : Product
  Product3 : Product
  Sum : Sum  Inputs=|+-
  Sum1 : Sum  Inputs=|++
  Sum2 : Sum  Inputs=|+---
  " G(t)" : Outport
  X(t) : Outport  Port=2
  I(t) : Outport  Port=3
  wires:
  Gain2/1 -> Sum1/1
  Gain/1 -> Sum/1
  " u(t)"/1 -> Gain/1
  Sum/1 -> Integrator/1
  Gain1/1 -> Sum/2
  Integrator2/1 -> Product3/2, " G(t)"/1, Gain5/1
  Integrator1/1 -> Product1/2, Gain3/1, X(t)/1
  Integrator/1 -> Gain2/1, I(t)/1, Gain1/1
  Gain3/1 -> Sum1/2
  Gain4/1 -> Sum2/1
  Gain5/1 -> Sum2/4
  p(t)/1 -> Gain4/1
  Sum1/1 -> Integrator1/1
  Sum2/1 -> Integrator2/1
  Constant/1 -> Product1/1
  Constant1/1 -> Product3/1
  Product3/1 -> Sum2/3
  Product1/1 -> Sum2/2

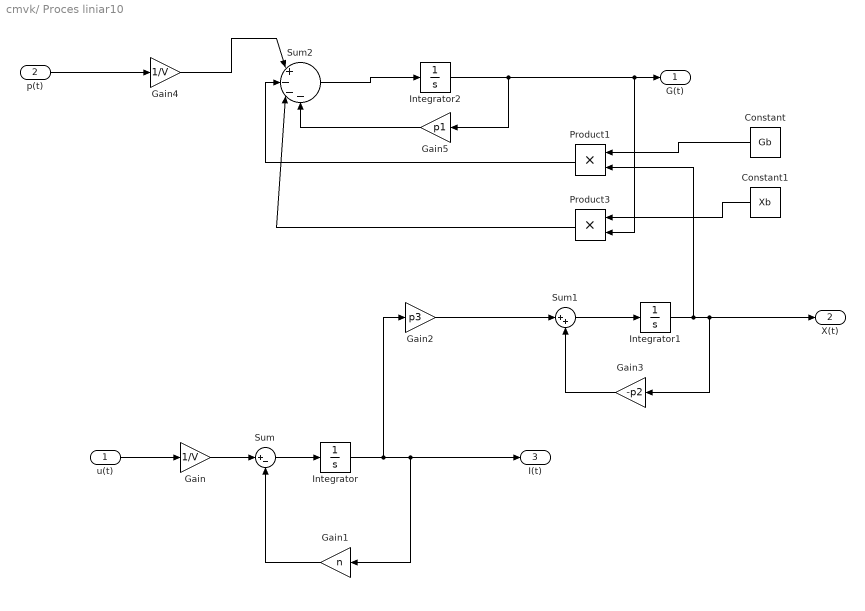
== system cmvk/ Proces liniar10 ==
  " u(t)" : Inport
  p(t) : Inport  Port=2
  Constant : Constant  Value=Gb
  Constant1 : Constant  Value=Xb
  Gain : Gain  Gain=1/V
  Gain1 : Gain  Gain=n
  Gain2 : Gain  Gain=p3
  Gain3 : Gain  Gain=-p2
  Gain4 : Gain  Gain=1/V
  Gain5 : Gain  Gain=p1
  Integrator : Integrator
  Integrator1 : Integrator
  Integrator2 : Integrator  InitialCondition=G0
  Product1 : Product
  Product3 : Product
  Sum : Sum  Inputs=|+-
  Sum1 : Sum  Inputs=|++
  Sum2 : Sum  Inputs=|+---
  " G(t)" : Outport
  X(t) : Outport  Port=2
  I(t) : Outport  Port=3
  wires:
  Gain2/1 -> Sum1/1
  Gain/1 -> Sum/1
  " u(t)"/1 -> Gain/1
  Sum/1 -> Integrator/1
  Gain1/1 -> Sum/2
  Integrator2/1 -> Product3/2, " G(t)"/1, Gain5/1
  Integrator1/1 -> Product1/2, Gain3/1, X(t)/1
  Integrator/1 -> Gain2/1, I(t)/1, Gain1/1
  Gain3/1 -> Sum1/2
  Gain4/1 -> Sum2/1
  Gain5/1 -> Sum2/4
  p(t)/1 -> Gain4/1
  Sum1/1 -> Integrator1/1
  Sum2/1 -> Integrator2/1
  Constant/1 -> Product1/1
  Constant1/1 -> Product3/1
  Product3/1 -> Sum2/3
  Product1/1 -> Sum2/2

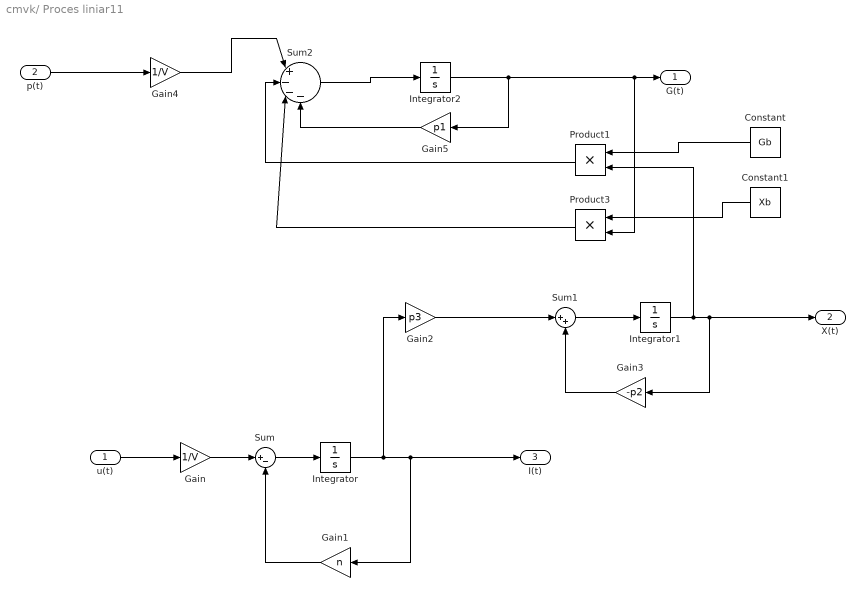
== system cmvk/ Proces liniar11 ==
  " u(t)" : Inport
  p(t) : Inport  Port=2
  Constant : Constant  Value=Gb
  Constant1 : Constant  Value=Xb
  Gain : Gain  Gain=1/V
  Gain1 : Gain  Gain=n
  Gain2 : Gain  Gain=p3
  Gain3 : Gain  Gain=-p2
  Gain4 : Gain  Gain=1/V
  Gain5 : Gain  Gain=p1
  Integrator : Integrator
  Integrator1 : Integrator
  Integrator2 : Integrator  InitialCondition=G0
  Product1 : Product
  Product3 : Product
  Sum : Sum  Inputs=|+-
  Sum1 : Sum  Inputs=|++
  Sum2 : Sum  Inputs=|+---
  " G(t)" : Outport
  X(t) : Outport  Port=2
  I(t) : Outport  Port=3
  wires:
  Gain2/1 -> Sum1/1
  Gain/1 -> Sum/1
  " u(t)"/1 -> Gain/1
  Sum/1 -> Integrator/1
  Gain1/1 -> Sum/2
  Integrator2/1 -> Product3/2, " G(t)"/1, Gain5/1
  Integrator1/1 -> Product1/2, Gain3/1, X(t)/1
  Integrator/1 -> Gain2/1, I(t)/1, Gain1/1
  Gain3/1 -> Sum1/2
  Gain4/1 -> Sum2/1
  Gain5/1 -> Sum2/4
  p(t)/1 -> Gain4/1
  Sum1/1 -> Integrator1/1
  Sum2/1 -> Integrator2/1
  Constant/1 -> Product1/1
  Constant1/1 -> Product3/1
  Product3/1 -> Sum2/3
  Product1/1 -> Sum2/2

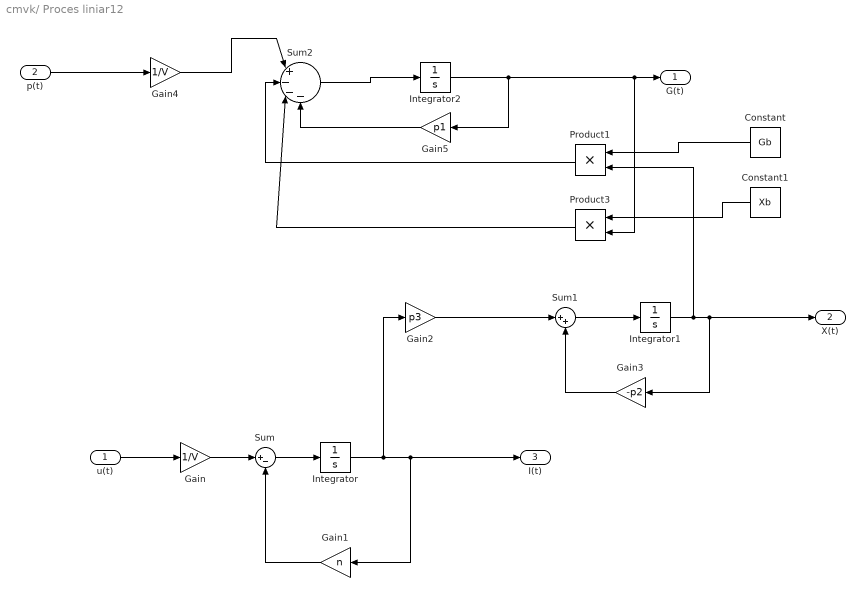
== system cmvk/ Proces liniar12 ==
  " u(t)" : Inport
  p(t) : Inport  Port=2
  Constant : Constant  Value=Gb
  Constant1 : Constant  Value=Xb
  Gain : Gain  Gain=1/V
  Gain1 : Gain  Gain=n
  Gain2 : Gain  Gain=p3
  Gain3 : Gain  Gain=-p2
  Gain4 : Gain  Gain=1/V
  Gain5 : Gain  Gain=p1
  Integrator : Integrator
  Integrator1 : Integrator
  Integrator2 : Integrator  InitialCondition=G0
  Product1 : Product
  Product3 : Product
  Sum : Sum  Inputs=|+-
  Sum1 : Sum  Inputs=|++
  Sum2 : Sum  Inputs=|+---
  " G(t)" : Outport
  X(t) : Outport  Port=2
  I(t) : Outport  Port=3
  wires:
  Gain2/1 -> Sum1/1
  Gain/1 -> Sum/1
  " u(t)"/1 -> Gain/1
  Sum/1 -> Integrator/1
  Gain1/1 -> Sum/2
  Integrator2/1 -> Product3/2, " G(t)"/1, Gain5/1
  Integrator1/1 -> Product1/2, Gain3/1, X(t)/1
  Integrator/1 -> Gain2/1, I(t)/1, Gain1/1
  Gain3/1 -> Sum1/2
  Gain4/1 -> Sum2/1
  Gain5/1 -> Sum2/4
  p(t)/1 -> Gain4/1
  Sum1/1 -> Integrator1/1
  Sum2/1 -> Integrator2/1
  Constant/1 -> Product1/1
  Constant1/1 -> Product3/1
  Product3/1 -> Sum2/3
  Product1/1 -> Sum2/2

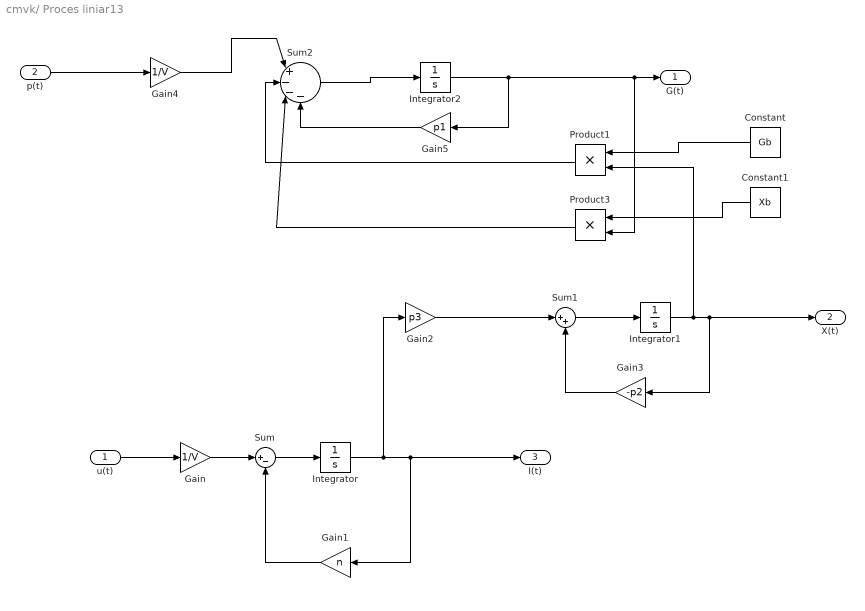
== system cmvk/ Proces liniar13 ==
  " u(t)" : Inport
  p(t) : Inport  Port=2
  Constant : Constant  Value=Gb
  Constant1 : Constant  Value=Xb
  Gain : Gain  Gain=1/V
  Gain1 : Gain  Gain=n
  Gain2 : Gain  Gain=p3
  Gain3 : Gain  Gain=-p2
  Gain4 : Gain  Gain=1/V
  Gain5 : Gain  Gain=p1
  Integrator : Integrator
  Integrator1 : Integrator
  Integrator2 : Integrator  InitialCondition=G0
  Product1 : Product
  Product3 : Product
  Sum : Sum  Inputs=|+-
  Sum1 : Sum  Inputs=|++
  Sum2 : Sum  Inputs=|+---
  " G(t)" : Outport
  X(t) : Outport  Port=2
  I(t) : Outport  Port=3
  wires:
  Gain2/1 -> Sum1/1
  Gain/1 -> Sum/1
  " u(t)"/1 -> Gain/1
  Sum/1 -> Integrator/1
  Gain1/1 -> Sum/2
  Integrator2/1 -> Product3/2, " G(t)"/1, Gain5/1
  Integrator1/1 -> Product1/2, Gain3/1, X(t)/1
  Integrator/1 -> Gain2/1, I(t)/1, Gain1/1
  Gain3/1 -> Sum1/2
  Gain4/1 -> Sum2/1
  Gain5/1 -> Sum2/4
  p(t)/1 -> Gain4/1
  Sum1/1 -> Integrator1/1
  Sum2/1 -> Integrator2/1
  Constant/1 -> Product1/1
  Constant1/1 -> Product3/1
  Product3/1 -> Sum2/3
  Product1/1 -> Sum2/2

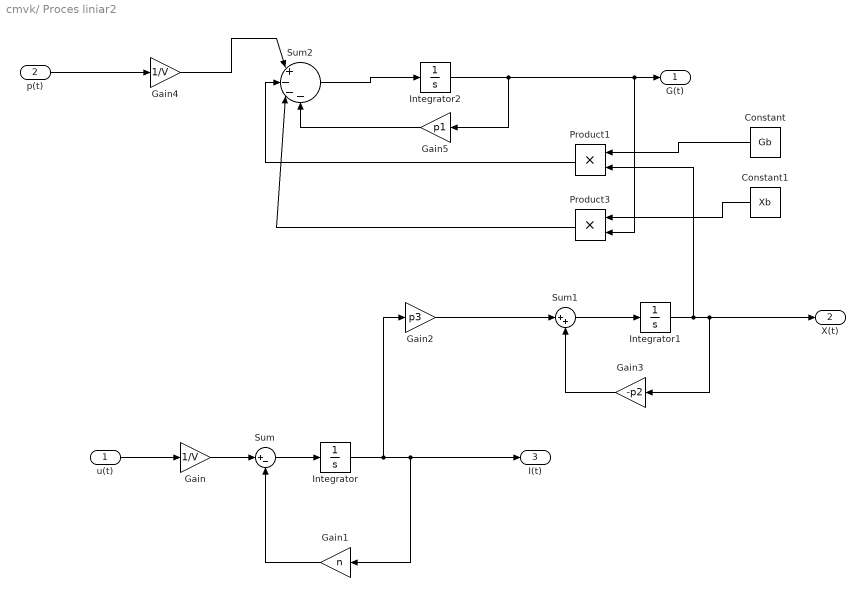
== system cmvk/ Proces liniar2 ==
  " u(t)" : Inport
  p(t) : Inport  Port=2
  Constant : Constant  Value=Gb
  Constant1 : Constant  Value=Xb
  Gain : Gain  Gain=1/V
  Gain1 : Gain  Gain=n
  Gain2 : Gain  Gain=p3
  Gain3 : Gain  Gain=-p2
  Gain4 : Gain  Gain=1/V
  Gain5 : Gain  Gain=p1
  Integrator : Integrator
  Integrator1 : Integrator
  Integrator2 : Integrator  InitialCondition=G0
  Product1 : Product
  Product3 : Product
  Sum : Sum  Inputs=|+-
  Sum1 : Sum  Inputs=|++
  Sum2 : Sum  Inputs=|+---
  " G(t)" : Outport
  X(t) : Outport  Port=2
  I(t) : Outport  Port=3
  wires:
  Gain2/1 -> Sum1/1
  Gain/1 -> Sum/1
  " u(t)"/1 -> Gain/1
  Sum/1 -> Integrator/1
  Gain1/1 -> Sum/2
  Integrator2/1 -> Product3/2, " G(t)"/1, Gain5/1
  Integrator1/1 -> Product1/2, Gain3/1, X(t)/1
  Integrator/1 -> Gain2/1, I(t)/1, Gain1/1
  Gain3/1 -> Sum1/2
  Gain4/1 -> Sum2/1
  Gain5/1 -> Sum2/4
  p(t)/1 -> Gain4/1
  Sum1/1 -> Integrator1/1
  Sum2/1 -> Integrator2/1
  Constant/1 -> Product1/1
  Constant1/1 -> Product3/1
  Product3/1 -> Sum2/3
  Product1/1 -> Sum2/2

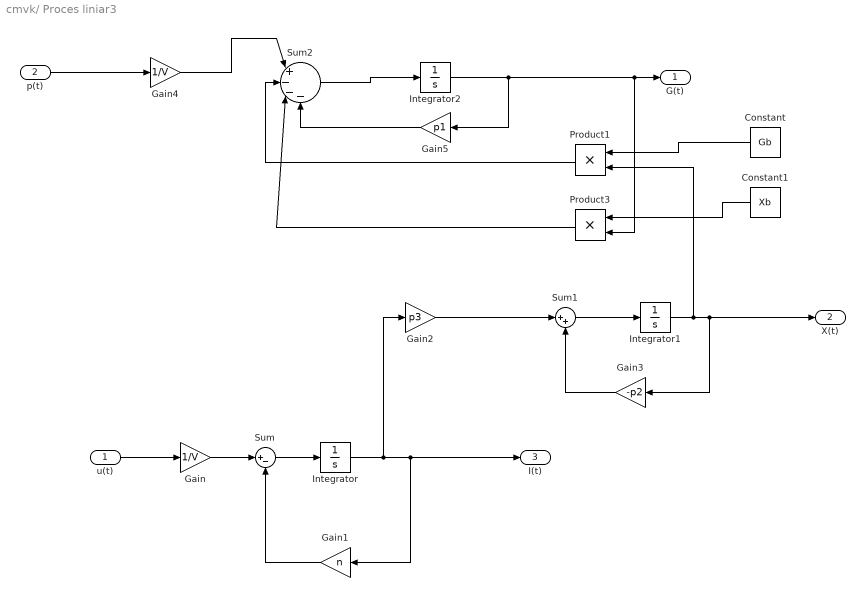
== system cmvk/ Proces liniar3 ==
  " u(t)" : Inport
  p(t) : Inport  Port=2
  Constant : Constant  Value=Gb
  Constant1 : Constant  Value=Xb
  Gain : Gain  Gain=1/V
  Gain1 : Gain  Gain=n
  Gain2 : Gain  Gain=p3
  Gain3 : Gain  Gain=-p2
  Gain4 : Gain  Gain=1/V
  Gain5 : Gain  Gain=p1
  Integrator : Integrator
  Integrator1 : Integrator
  Integrator2 : Integrator  InitialCondition=G0
  Product1 : Product
  Product3 : Product
  Sum : Sum  Inputs=|+-
  Sum1 : Sum  Inputs=|++
  Sum2 : Sum  Inputs=|+---
  " G(t)" : Outport
  X(t) : Outport  Port=2
  I(t) : Outport  Port=3
  wires:
  Gain2/1 -> Sum1/1
  Gain/1 -> Sum/1
  " u(t)"/1 -> Gain/1
  Sum/1 -> Integrator/1
  Gain1/1 -> Sum/2
  Integrator2/1 -> Product3/2, " G(t)"/1, Gain5/1
  Integrator1/1 -> Product1/2, Gain3/1, X(t)/1
  Integrator/1 -> Gain2/1, I(t)/1, Gain1/1
  Gain3/1 -> Sum1/2
  Gain4/1 -> Sum2/1
  Gain5/1 -> Sum2/4
  p(t)/1 -> Gain4/1
  Sum1/1 -> Integrator1/1
  Sum2/1 -> Integrator2/1
  Constant/1 -> Product1/1
  Constant1/1 -> Product3/1
  Product3/1 -> Sum2/3
  Product1/1 -> Sum2/2

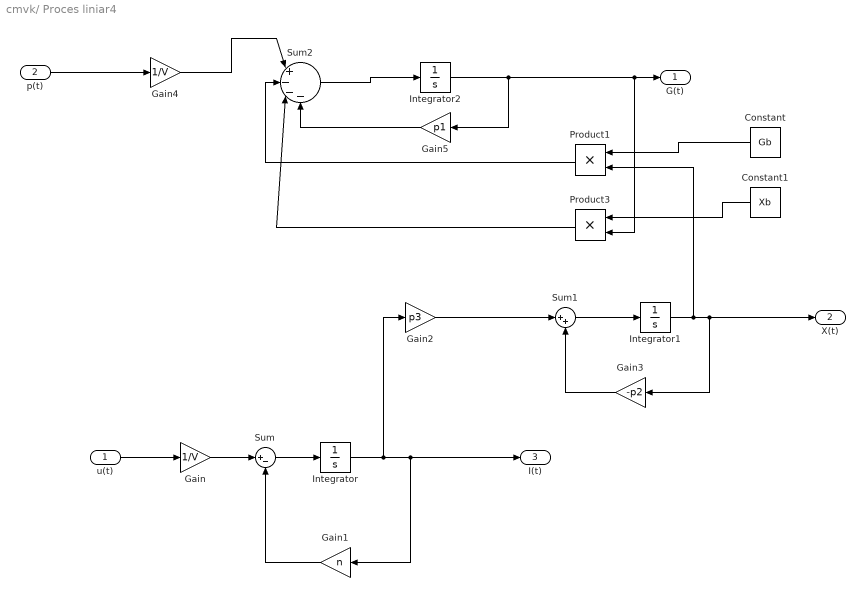
== system cmvk/ Proces liniar4 ==
  " u(t)" : Inport
  p(t) : Inport  Port=2
  Constant : Constant  Value=Gb
  Constant1 : Constant  Value=Xb
  Gain : Gain  Gain=1/V
  Gain1 : Gain  Gain=n
  Gain2 : Gain  Gain=p3
  Gain3 : Gain  Gain=-p2
  Gain4 : Gain  Gain=1/V
  Gain5 : Gain  Gain=p1
  Integrator : Integrator
  Integrator1 : Integrator
  Integrator2 : Integrator  InitialCondition=G0
  Product1 : Product
  Product3 : Product
  Sum : Sum  Inputs=|+-
  Sum1 : Sum  Inputs=|++
  Sum2 : Sum  Inputs=|+---
  " G(t)" : Outport
  X(t) : Outport  Port=2
  I(t) : Outport  Port=3
  wires:
  Gain2/1 -> Sum1/1
  Gain/1 -> Sum/1
  " u(t)"/1 -> Gain/1
  Sum/1 -> Integrator/1
  Gain1/1 -> Sum/2
  Integrator2/1 -> Product3/2, " G(t)"/1, Gain5/1
  Integrator1/1 -> Product1/2, Gain3/1, X(t)/1
  Integrator/1 -> Gain2/1, I(t)/1, Gain1/1
  Gain3/1 -> Sum1/2
  Gain4/1 -> Sum2/1
  Gain5/1 -> Sum2/4
  p(t)/1 -> Gain4/1
  Sum1/1 -> Integrator1/1
  Sum2/1 -> Integrator2/1
  Constant/1 -> Product1/1
  Constant1/1 -> Product3/1
  Product3/1 -> Sum2/3
  Product1/1 -> Sum2/2

== system cmvk/perturbatie1 ==
  Clock : Clock
  Constant : Constant  Value=Dg
  Constant1 : Constant  Value=Ag
  Gain : Gain  Gain=-1/tg_max
  Gain1 : Gain  Gain=1/(tg_max*tg_max)
  Math Function : Math
  Product : Product  Inputs=4
  p(t) : Outport
  wires:
  Constant/1 -> Product/1
  Constant1/1 -> Product/2
  Clock/1 -> Gain/1, Product/3
  Gain/1 -> Math Function/1
  Math Function/1 -> Product/4
  Product/1 -> Gain1/1
  Gain1/1 -> p(t)/1

== system cmvk/perturbatie10 ==
  Clock : Clock
  Constant : Constant  Value=Dg
  Constant1 : Constant  Value=Ag
  Gain : Gain  Gain=-1/tg_max
  Gain1 : Gain  Gain=1/(tg_max*tg_max)
  Math Function : Math
  Product : Product  Inputs=4
  p(t) : Outport
  wires:
  Constant/1 -> Product/1
  Constant1/1 -> Product/2
  Clock/1 -> Gain/1, Product/3
  Gain/1 -> Math Function/1
  Math Function/1 -> Product/4
  Product/1 -> Gain1/1
  Gain1/1 -> p(t)/1

== system cmvk/perturbatie11 ==
  Clock : Clock
  Constant : Constant  Value=Dg
  Constant1 : Constant  Value=Ag
  Gain : Gain  Gain=-1/tg_max
  Gain1 : Gain  Gain=1/(tg_max*tg_max)
  Math Function : Math
  Product : Product  Inputs=4
  p(t) : Outport
  wires:
  Constant/1 -> Product/1
  Constant1/1 -> Product/2
  Clock/1 -> Gain/1, Product/3
  Gain/1 -> Math Function/1
  Math Function/1 -> Product/4
  Product/1 -> Gain1/1
  Gain1/1 -> p(t)/1

== system cmvk/perturbatie12 ==
  Clock : Clock
  Constant : Constant  Value=Dg
  Constant1 : Constant  Value=Ag
  Gain : Gain  Gain=-1/tg_max
  Gain1 : Gain  Gain=1/(tg_max*tg_max)
  Math Function : Math
  Product : Product  Inputs=4
  p(t) : Outport
  wires:
  Constant/1 -> Product/1
  Constant1/1 -> Product/2
  Clock/1 -> Gain/1, Product/3
  Gain/1 -> Math Function/1
  Math Function/1 -> Product/4
  Product/1 -> Gain1/1
  Gain1/1 -> p(t)/1

== system cmvk/perturbatie2 ==
  Clock : Clock
  Constant : Constant  Value=Dg
  Constant1 : Constant  Value=Ag
  Gain : Gain  Gain=-1/tg_max
  Gain1 : Gain  Gain=1/(tg_max*tg_max)
  Math Function : Math
  Product : Product  Inputs=4
  p(t) : Outport
  wires:
  Constant/1 -> Product/1
  Constant1/1 -> Product/2
  Clock/1 -> Gain/1, Product/3
  Gain/1 -> Math Function/1
  Math Function/1 -> Product/4
  Product/1 -> Gain1/1
  Gain1/1 -> p(t)/1

== system cmvk/perturbatie3 ==
  Clock : Clock
  Constant : Constant  Value=Dg
  Constant1 : Constant  Value=Ag
  Gain : Gain  Gain=-1/tg_max
  Gain1 : Gain  Gain=1/(tg_max*tg_max)
  Math Function : Math
  Product : Product  Inputs=4
  p(t) : Outport
  wires:
  Constant/1 -> Product/1
  Constant1/1 -> Product/2
  Clock/1 -> Gain/1, Product/3
  Gain/1 -> Math Function/1
  Math Function/1 -> Product/4
  Product/1 -> Gain1/1
  Gain1/1 -> p(t)/1

== system cmvk/perturbatie37 ==
  Clock : Clock
  Constant : Constant  Value=Dg
  Constant1 : Constant  Value=Ag
  Gain : Gain  Gain=-1/tg_max
  Gain1 : Gain  Gain=1/(tg_max*tg_max)
  Math Function : Math
  Product : Product  Inputs=4
  p(t) : Outport
  wires:
  Constant/1 -> Product/1
  Constant1/1 -> Product/2
  Clock/1 -> Gain/1, Product/3
  Gain/1 -> Math Function/1
  Math Function/1 -> Product/4
  Product/1 -> Gain1/1
  Gain1/1 -> p(t)/1

== system cmvk/perturbatie4 ==
  Clock : Clock
  Constant : Constant  Value=Dg
  Constant1 : Constant  Value=Ag
  Gain : Gain  Gain=-1/tg_max
  Gain1 : Gain  Gain=1/(tg_max*tg_max)
  Math Function : Math
  Product : Product  Inputs=4
  p(t) : Outport
  wires:
  Constant/1 -> Product/1
  Constant1/1 -> Product/2
  Clock/1 -> Gain/1, Product/3
  Gain/1 -> Math Function/1
  Math Function/1 -> Product/4
  Product/1 -> Gain1/1
  Gain1/1 -> p(t)/1

== system cmvk/perturbatie5 ==
  Clock : Clock
  Constant : Constant  Value=Dg
  Constant1 : Constant  Value=Ag
  Gain : Gain  Gain=-1/tg_max
  Gain1 : Gain  Gain=1/(tg_max*tg_max)
  Math Function : Math
  Product : Product  Inputs=4
  p(t) : Outport
  wires:
  Constant/1 -> Product/1
  Constant1/1 -> Product/2
  Clock/1 -> Gain/1, Product/3
  Gain/1 -> Math Function/1
  Math Function/1 -> Product/4
  Product/1 -> Gain1/1
  Gain1/1 -> p(t)/1

== system cmvk/perturbatie6 ==
  Clock : Clock
  Constant : Constant  Value=Dg
  Constant1 : Constant  Value=Ag
  Gain : Gain  Gain=-1/tg_max
  Gain1 : Gain  Gain=1/(tg_max*tg_max)
  Math Function : Math
  Product : Product  Inputs=4
  p(t) : Outport
  wires:
  Constant/1 -> Product/1
  Constant1/1 -> Product/2
  Clock/1 -> Gain/1, Product/3
  Gain/1 -> Math Function/1
  Math Function/1 -> Product/4
  Product/1 -> Gain1/1
  Gain1/1 -> p(t)/1

== system cmvk/perturbatie7 ==
  Clock : Clock
  Constant : Constant  Value=Dg
  Constant1 : Constant  Value=Ag
  Gain : Gain  Gain=-1/tg_max
  Gain1 : Gain  Gain=1/(tg_max*tg_max)
  Math Function : Math
  Product : Product  Inputs=4
  p(t) : Outport
  wires:
  Constant/1 -> Product/1
  Constant1/1 -> Product/2
  Clock/1 -> Gain/1, Product/3
  Gain/1 -> Math Function/1
  Math Function/1 -> Product/4
  Product/1 -> Gain1/1
  Gain1/1 -> p(t)/1

== system cmvk/perturbatie8 ==
  Clock : Clock
  Constant : Constant  Value=Dg
  Constant1 : Constant  Value=Ag
  Gain : Gain  Gain=-1/tg_max
  Gain1 : Gain  Gain=1/(tg_max*tg_max)
  Math Function : Math
  Product : Product  Inputs=4
  p(t) : Outport
  wires:
  Constant/1 -> Product/1
  Constant1/1 -> Product/2
  Clock/1 -> Gain/1, Product/3
  Gain/1 -> Math Function/1
  Math Function/1 -> Product/4
  Product/1 -> Gain1/1
  Gain1/1 -> p(t)/1

== system cmvk/perturbatie9 ==
  Clock : Clock
  Constant : Constant  Value=Dg
  Constant1 : Constant  Value=Ag
  Gain : Gain  Gain=-1/tg_max
  Gain1 : Gain  Gain=1/(tg_max*tg_max)
  Math Function : Math
  Product : Product  Inputs=4
  p(t) : Outport
  wires:
  Constant/1 -> Product/1
  Constant1/1 -> Product/2
  Clock/1 -> Gain/1, Product/3
  Gain/1 -> Math Function/1
  Math Function/1 -> Product/4
  Product/1 -> Gain1/1
  Gain1/1 -> p(t)/1
